simulink library "inp"  (R2021b)
settings: Solver=VariableStepAuto  StartTime=0.0  StopTime=10.0  RelTol=1e-3
undefined symbols (not defined in the file): C_TASK_5MS_S, FALSE, KINP_AcoreReadyToSlp_flg_ovrdflg, KINP_AcoreReadyToSlp_flg_ovrdval, KINP_AllowMovThd_OTA_enum_ovrdflg, KINP_AllowMovThd_OTA_enum_ovrdval, KINP_APSAngleTarget_Deg_ovrdflg, KINP_APSAngleTarget_Deg_ovrdval, KINP_APSDecReq_mps2_ovrdflg, KINP_APSDecReq_mps2_ovrdval, KINP_APSDecReqA_flg_ovrdflg, KINP_APSDecReqA_flg_ovrdval, KINP_APSDFLL_cm_ovrdflg, KINP_APSDFLL_cm_ovrdval, KINP_APSDFLR_cm_ovrdflg, KINP_APSDFLR_cm_ovrdval, KINP_APSDRLL_cm_ovrdflg, KINP_APSDRLL_cm_ovrdval, KINP_APSDRLR_cm_ovrdflg, KINP_APSDRLR_cm_ovrdval, KINP_APSExitCondition_enum_ovrdflg, KINP_APSExitCondition_enum_ovrdval, KINP_APSHWVer_enum_ovrdflg, KINP_APSHWVer_enum_ovrdval, KINP_APSProgressPCT_pct_ovrdflg, KINP_APSProgressPCT_pct_ovrdval, KINP_APSReq_enum_ovrdflg, KINP_APSReq_enum_ovrdval, KINP_APSRQDisplay_enum_ovrdflg, KINP_APSRQDisplay_enum_ovrdval, KINP_APSRqEPASCtrl_flg_ovrdflg, KINP_APSRqEPASCtrl_flg_ovrdval, KINP_APSShiftPosnReq_enum_ovrdval, KINP_APSShiftPosnReq_enum_ovrflg, KINP_APSSpeedCMD_kph_ovrdval, KINP_APSSpeedCMD_kph_ovrflg, KINP_APSStaSystem_enum_ovrdflg, KINP_APSStaSystem_enum_ovrdval, KINP_APSSWVer_enum_ovrdflg, KINP_APSSWVer_enum_ovrdval, KINP_APSVMCReqA_flg_ovrdval, KINP_APSVMCReqA_flg_ovrflg, KINP_APSVRqEPASCtrl_flg_ovrdflg, KINP_APSVRqEPASCtrl_flg_ovrdval, KINP_AuxBattVolmV_mV_ovrdflg, KINP_AuxBattVolmV_mV_ovrdval, KINP_CAASSta_enum_ovrdflg, KINP_CAASSta_enum_ovrdval, KINP_CAASVMCReqA_flg_ovrdval, KINP_CAASVMCReqA_flg_ovrflg, KINP_Chime_enum_ovrdflg, KINP_Chime_enum_ovrdval, KINP_ClearDTCcmd_flg_ovrdflg, KINP_ClearDTCcmd_flg_ovrdval, KINP_EvccAplusPwrUpReq_flg_ovrdflg, KINP_EvccAplusPwrUpReq_flg_ovrdval, KINP_LFID_raw_ovrdval, KINP_LFID_raw_ovrflg, KINP_LRID_raw_ovrdval, KINP_MemOffsetAccX_raw16_ovrdflg ... (+118)
libraries: FVT_lib x595, hcu_lib x1
(part 6 of 27)

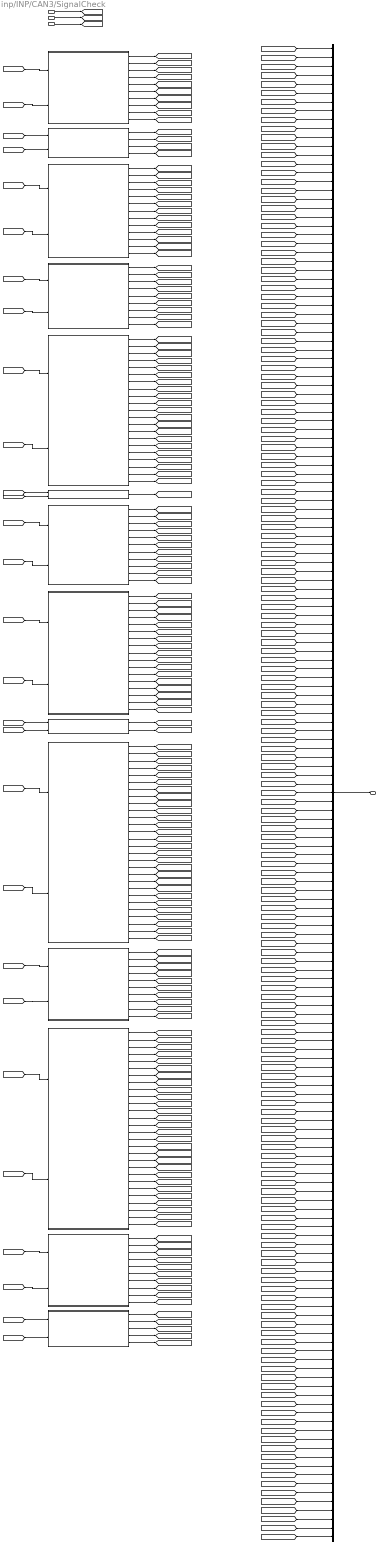
== system inp/INP/CAN3/SignalCheck ==
  inp_CanValid_bus : Inport
  TASK_TIME_S : Inport  Port=2
  BHAL_outputs : Inport  Port=3
  BMS1 : Subsystem
  BMS2 : Subsystem
  BMS3 : Subsystem
  BMS4 : Subsystem
  BMS6 : Subsystem
  BMS7 : Subsystem
  CCU1 : Subsystem
  CCU2 : Subsystem
  CCU4 : Subsystem
  MCU_F1 : Subsystem
  MCU_F2 : Subsystem
  MCU_R1 : Subsystem
  MCU_R2 : Subsystem
  Shifter1 : Subsystem
  bus_creator : BusCreator  Inputs=169
  inp_Hal_bus : Outport
  wires:
  inp_CanValid_bus/1 -> [inp_CanValid_bus]
  TASK_TIME_S/1 -> [TASK_TIME_S]
  BHAL_outputs/1 -> [BHAL_outputs]
  [BHAL_outputs] -> BMS1/1(BHAL_outputs)
  [inp_CanValid_bus] -> BMS1/2(inp_CanValid_bus)
  BMS1/1(VINP_BMS1CSErr_flg) -> [VINP_BMS1CSErr_flg]
  BMS1/2(VINP_BMS1RCErr_flg) -> [VINP_BMS1RCErr_flg]
  BMS1/3(VINP_BMSChckSum1_enum) -> [VINP_BMSChckSum1_enum]
  BMS1/4(VINP_BMSRolCnct1_enum) -> [VINP_BMSRolCnct1_enum]
  BMS1/5(VINP_HVBPwrAvailChrg_kW) -> [VINP_HVBPwrAvailChrg_kW]
  BMS1/6(VINP_HVBPwrAvailChrg30_kW) -> [VINP_HVBPwrAvailChrg30_kW]
  BMS1/7(VINP_HVBPwrAvailChrg60_kW) -> [VINP_HVBPwrAvailChrg60_kW]
  BMS1/8(VINP_HVBPwrAvailDchrg_kW) -> [VINP_HVBPwrAvailDchrg_kW]
  BMS1/9(VINP_HVBPwrAvailDchrg30_kW) -> [VINP_HVBPwrAvailDchrg30_kW]
  BMS1/10(VINP_HVBPwrAvailDchrg60_kW) -> [VINP_HVBPwrAvailDchrg60_kW]
  [BHAL_outputs] -> BMS2/1(BHAL_outputs)
  [inp_CanValid_bus] -> BMS2/2(inp_CanValid_bus)
  BMS2/1(VINP_HVInVolt_V) -> [VINP_HVInVolt_V]
  BMS2/2(VINP_LVBattDet12V_V) -> [VINP_LVBattDet12V_V]
  BMS2/3(VINP_OBCDCCurLm_A) -> [VINP_OBCDCCurLm_A]
  BMS2/4(VINP_OBCDCVoltLm_V) -> [VINP_OBCDCVoltLm_V]
  [BHAL_outputs] -> BMS3/1(BHAL_outputs)
  [inp_CanValid_bus] -> BMS3/2(inp_CanValid_bus)
  BMS3/1(VINP_ACChrgCurrDis_A) -> [VINP_ACChrgCurrDis_A]
  BMS3/2(VINP_HVBChrgPwr_kWh) -> [VINP_HVBChrgPwr_kWh]
  BMS3/3(VINP_HVBChrgPwrTotal_kWh) -> [VINP_HVBChrgPwrTotal_kWh]
  BMS3/4(VINP_HVBDrvPwr_kWh) -> [VINP_HVBDrvPwr_kWh]
  BMS3/5(VINP_HVBDrvPwrTotal_kWh) -> [VINP_HVBDrvPwrTotal_kWh]
  BMS3/6(VINP_HVBFullChrgPwr_kWh) -> [VINP_HVBFullChrgPwr_kWh]
  BMS3/7(VINP_HVBIsoImpedenceN_Megaohm) -> [VINP_HVBIsoImpedenceN_Megaohm]
  BMS3/8(VINP_HVBIsoImpedenceP_Megaohm) -> [VINP_HVBIsoImpedenceP_Megaohm]
  BMS3/9(VINP_HVBSOH_pct) -> [VINP_HVBSOH_pct]
  BMS3/10(VINP_HVBattPackVolt_V) -> [VINP_HVBattPackVolt_V]
  BMS3/11(VINP_HVBattSOC_pct) -> [VINP_HVBattSOC_pct]
  BMS3/12(VINP_HVBattSOCDis_pct) -> [VINP_HVBattSOCDis_pct]
  BMS3/13(VINP_RemainChrgTime_min) -> [VINP_RemainChrgTime_min]
  [BHAL_outputs] -> BMS4/1(BHAL_outputs)
  [inp_CanValid_bus] -> BMS4/2(inp_CanValid_bus)
  BMS4/1(VINP_CellTempAvg_C) -> [VINP_CellTempAvg_C]
  BMS4/2(VINP_HVBCellVoltMax_mV) -> [VINP_HVBCellVoltMax_mV]
  BMS4/3(VINP_HVBCellVoltMin_mV) -> [VINP_HVBCellVoltMin_mV]
  BMS4/4(VINP_HVBMTempMax_C) -> [VINP_HVBMTempMax_C]
  BMS4/5(VINP_HVBMTempMin_C) -> [VINP_HVBMTempMin_C]
  BMS4/6(VINP_MaxCellTempNum_enum) -> [VINP_MaxCellTempNum_enum]
  BMS4/7(VINP_MaxCellVoltNum_enum) -> [VINP_MaxCellVoltNum_enum]
  BMS4/8(VINP_MinCellTempNum_enum) -> [VINP_MinCellTempNum_enum]
  BMS4/9(VINP_MinCellVoltNum_enum) -> [VINP_MinCellVoltNum_enum]
  [BHAL_outputs] -> BMS6/1(BHAL_outputs)
  [inp_CanValid_bus] -> BMS6/2(inp_CanValid_bus)
  BMS6/1(VINP_BMS6CSErr_flg) -> [VINP_BMS6CSErr_flg]
  BMS6/2(VINP_BMS6RCErr_flg) -> [VINP_BMS6RCErr_flg]
  BMS6/3(VINP_BMSChckSum_enum) -> [VINP_BMSChckSum_enum]
  BMS6/4(VINP_BMSRolCnct_enum) -> [VINP_BMSRolCnct_enum]
  BMS6/5(VINP_BMSREADY_flg) -> [VINP_BMSREADY_flg]
  BMS6/6(VINP_BMSWarn1_flg) -> [VINP_BMSWarn1_flg]
  BMS6/7(VINP_BMSWarn2_flg) -> [VINP_BMSWarn2_flg]
  BMS6/8(VINP_BMSWarn3_flg) -> [VINP_BMSWarn3_flg]
  BMS6/9(VINP_BMSWarn4_flg) -> [VINP_BMSWarn4_flg]
  BMS6/10(VINP_BMSWarn5_flg) -> [VINP_BMSWarn5_flg]
  BMS6/11(VINP_BMSWarn6_flg) -> [VINP_BMSWarn6_flg]
  BMS6/12(VINP_BMSWarn7_flg) -> [VINP_BMSWarn7_flg]
  BMS6/13(VINP_BMSWarn8_flg) -> [VINP_BMSWarn8_flg]
  BMS6/14(VINP_ChrgPlugSta_enum) -> [VINP_ChrgPlugSta_enum]
  BMS6/15(VINP_ExtChrgSta_enum) -> [VINP_ExtChrgSta_enum]
  BMS6/16(VINP_HVBContactorSta_flg) -> [VINP_HVBContactorSta_flg]
  BMS6/17(VINP_HVBHVILErr_flg) -> [VINP_HVBHVILErr_flg]
  BMS6/18(VINP_HVBPreheatPrecoolSta_enum) -> [VINP_HVBPreheatPrecoolSta_enum]
  BMS6/19(VINP_HVBattReady4Pre_enum) -> [VINP_HVBattReady4Pre_enum]
  BMS6/20(VINP_HVILSta_flg) -> [VINP_HVILSta_flg]
  BMS6/21(VINP_V2LSta_enum) -> [VINP_V2LSta_enum]
  [BHAL_outputs] -> BMS7/1(BHAL_outputs)
  [inp_CanValid_bus] -> BMS7/2(inp_CanValid_bus)
  BMS7/1(VINP_HVBattErr_flg) -> [VINP_HVBattErr_flg]
  [BHAL_outputs] -> CCU1/1(BHAL_outputs)
  [inp_CanValid_bus] -> CCU1/2(inp_CanValid_bus)
  CCU1/1(VINP_CCU1CSErr_flg) -> [VINP_CCU1CSErr_flg]
  CCU1/2(VINP_CCU1RCErr_flg) -> [VINP_CCU1RCErr_flg]
  CCU1/3(VINP_CSCCU1_enum) -> [VINP_CSCCU1_enum]
  CCU1/4(VINP_DCDCAuxVolt_V) -> [VINP_DCDCAuxVolt_V]
  CCU1/5(VINP_DCDCInVoltInf_V) -> [VINP_DCDCInVoltInf_V]
  CCU1/6(VINP_DCDCPreCompleted_enum) -> [VINP_DCDCPreCompleted_enum]
  CCU1/7(VINP_OBCDCCurrInf_A) -> [VINP_OBCDCCurrInf_A]
  CCU1/8(VINP_OBCDCVoltInf_V) -> [VINP_OBCDCVoltInf_V]
  CCU1/9(VINP_OBCPreCompleted_enum) -> [VINP_OBCPreCompleted_enum]
  CCU1/10(VINP_OBCWakeup4Plugin_flg) -> [VINP_OBCWakeup4Plugin_flg]
  CCU1/11(VINP_RCCCU1_enum) -> [VINP_RCCCU1_enum]
  [BHAL_outputs] -> CCU2/1(BHAL_outputs)
  [inp_CanValid_bus] -> CCU2/2(inp_CanValid_bus)
  CCU2/1(VINP_CCU2CSErr_flg) -> [VINP_CCU2CSErr_flg]
  CCU2/2(VINP_CCU2RCErr_flg) -> [VINP_CCU2RCErr_flg]
  CCU2/3(VINP_CSCCU2_enum) -> [VINP_CSCCU2_enum]
  CCU2/4(VINP_DCDCEnaSta_flg) -> [VINP_DCDCEnaSta_flg]
  CCU2/5(VINP_DCDCFaultSta_enum) -> [VINP_DCDCFaultSta_enum]
  CCU2/6(VINP_DCDCReady4Pre_flg) -> [VINP_DCDCReady4Pre_flg]
  CCU2/7(VINP_DCDCTemp_C) -> [VINP_DCDCTemp_C]
  CCU2/8(VINP_OBCACCurrInf_A) -> [VINP_OBCACCurrInf_A]
  CCU2/9(VINP_OBCACVoltInf_V) -> [VINP_OBCACVoltInf_V]
  CCU2/10(VINP_OBCEnaSta_flg) -> [VINP_OBCEnaSta_flg]
  CCU2/11(VINP_OBCFaultSta_enum) -> [VINP_OBCFaultSta_enum]
  CCU2/12(VINP_OBCPluginSta_flg) -> [VINP_OBCPluginSta_flg]
  CCU2/13(VINP_OBCReady4Pre_flg) -> [VINP_OBCReady4Pre_flg]
  CCU2/14(VINP_OBCTemp_C) -> [VINP_OBCTemp_C]
  CCU2/15(VINP_OBCV2LSta_enum) -> [VINP_OBCV2LSta_enum]
  CCU2/16(VINP_OBCACCurLim_enum) -> [VINP_OBCACCurLim_enum]
  CCU2/17(VINP_RCCCU2_enum) -> [VINP_RCCCU2_enum]
  [BHAL_outputs] -> CCU4/1(BHAL_outputs)
  [inp_CanValid_bus] -> CCU4/2(inp_CanValid_bus)
  CCU4/1(VINP_DCDCAuxCur_A) -> [VINP_DCDCAuxCur_A]
  CCU4/2(VINP_DCDCHVCur_A) -> [VINP_DCDCHVCur_A]
  [BHAL_outputs] -> MCU_F1/1(BHAL_outputs)
  [inp_CanValid_bus] -> MCU_F1/2(inp_CanValid_bus)
  MCU_F1/1(VINP_MCUF1CSErr_flg) -> [VINP_MCUF1CSErr_flg]
  MCU_F1/2(VINP_MCUF1RCErr_flg) -> [VINP_MCUF1RCErr_flg]
  MCU_F1/3(VINP_FrActvDmpDisabSta_flg) -> [VINP_FrActvDmpDisabSta_flg]
  MCU_F1/4(VINP_FrEDUDrtSta_flg) -> [VINP_FrEDUDrtSta_flg]
  MCU_F1/5(VINP_FrEDUOpratingSta_flg) -> [VINP_FrEDUOpratingSta_flg]
  MCU_F1/6(VINP_FrEDURealTMTq_Nm) -> [VINP_FrEDURealTMTq_Nm]
  MCU_F1/7(VINP_FrEDURotateDirction_enum) -> [VINP_FrEDURotateDirction_enum]
  MCU_F1/8(VINP_FrEDUTqReqFbk_Nm) -> [VINP_FrEDUTqReqFbk_Nm]
  MCU_F1/9(VINP_FrMCU1Chksum_enum) -> [VINP_FrMCU1Chksum_enum]
  MCU_F1/10(VINP_FrMCU1RolCnt_enum) -> [VINP_FrMCU1RolCnt_enum]
  MCU_F1/11(VINP_FrMCUBAT_V) -> [VINP_FrMCUBAT_V]
  MCU_F1/12(VINP_FrMCUDCBusCurr_A) -> [VINP_FrMCUDCBusCurr_A]
  MCU_F1/13(VINP_FrMCUDCBusVolt_V) -> [VINP_FrMCUDCBusVolt_V]
  MCU_F1/14(VINP_FrMCUDischrgSta_flg) -> [VINP_FrMCUDischrgSta_flg]
  MCU_F1/15(VINP_FrMCUEnaSta_flg) -> [VINP_FrMCUEnaSta_flg]
  MCU_F1/16(VINP_FrMCUErr_enum) -> [VINP_FrMCUErr_enum]
  MCU_F1/17(VINP_FrMCUIGNsta_flg) -> [VINP_FrMCUIGNsta_flg]
  MCU_F1/18(VINP_FrMCUReady_flg) -> [VINP_FrMCUReady_flg]
  MCU_F1/19(VINP_FrMCUReady4Pre_flg) -> [VINP_FrMCUReady4Pre_flg]
  MCU_F1/20(VINP_FrMCUSysSta_enum) -> [VINP_FrMCUSysSta_enum]
  MCU_F1/21(VINP_FrMCUTemp_C) -> [VINP_FrMCUTemp_C]
  MCU_F1/22(VINP_FrMotorAvailTq_Nm) -> [VINP_FrMotorAvailTq_Nm]
  MCU_F1/23(VINP_FrRegenAvailTq_Nm) -> [VINP_FrRegenAvailTq_Nm]
  MCU_F1/24(VINP_FrTMSpd_rpm) -> [VINP_FrTMSpd_rpm]
  MCU_F1/25(VINP_FrTMTemp_C) -> [VINP_FrTMTemp_C]
  MCU_F1/26(VINP_FrTMid_A) -> [VINP_FrTMid_A]
  MCU_F1/27(VINP_FrTMiq_A) -> [VINP_FrTMiq_A]
  MCU_F1/28(VINP_MCUWarnF_enum) -> [VINP_MCUWarnF_enum]
  [BHAL_outputs] -> MCU_F2/1(BHAL_outputs)
  [inp_CanValid_bus] -> MCU_F2/2(inp_CanValid_bus)
  MCU_F2/1(VINP_FrCoolanttempReq_C) -> [VINP_FrCoolanttempReq_C]
  MCU_F2/2(VINP_FrEOPSpdSet_rpm) -> [VINP_FrEOPSpdSet_rpm]
  MCU_F2/3(VINP_FrFailcode1_enum) -> [VINP_FrFailcode1_enum]
  MCU_F2/4(VINP_FrFailcode2_enum) -> [VINP_FrFailcode2_enum]
  MCU_F2/5(VINP_FrFailcodehistory1_enum) -> [VINP_FrFailcodehistory1_enum]
  MCU_F2/6(VINP_FrFailcodehistory2_enum) -> [VINP_FrFailcodehistory2_enum]
  MCU_F2/7(VINP_FrLLCTemp_C) -> [VINP_FrLLCTemp_C]
  MCU_F2/8(VINP_FrLLCflowReq_Lpmin) -> [VINP_FrLLCflowReq_Lpmin]
  MCU_F2/9(VINP_FrMCUTempWarn_enum) -> [VINP_FrMCUTempWarn_enum]
  MCU_F2/10(VINP_FrTMTempWarn_enum) -> [VINP_FrTMTempWarn_enum]
  [BHAL_outputs] -> MCU_R1/1(BHAL_outputs)
  [inp_CanValid_bus] -> MCU_R1/2(inp_CanValid_bus)
  MCU_R1/1(VINP_MCUR1CSErr_flg) -> [VINP_MCUR1CSErr_flg]
  MCU_R1/2(VINP_MCUR1RCErr_flg) -> [VINP_MCUR1RCErr_flg]
  MCU_R1/3(VINP_MCUWarnR_enum) -> [VINP_MCUWarnR_enum]
  MCU_R1/4(VINP_RrActvDmpDisabSta_flg) -> [VINP_RrActvDmpDisabSta_flg]
  MCU_R1/5(VINP_RrEDUDrtSta_flg) -> [VINP_RrEDUDrtSta_flg]
  MCU_R1/6(VINP_RrEDUOpratingSta_flg) -> [VINP_RrEDUOpratingSta_flg]
  MCU_R1/7(VINP_RrEDURealTMTq_Nm) -> [VINP_RrEDURealTMTq_Nm]
  MCU_R1/8(VINP_RrEDURotateDirction_enum) -> [VINP_RrEDURotateDirction_enum]
  MCU_R1/9(VINP_RrEDUTqReqFbk_Nm) -> [VINP_RrEDUTqReqFbk_Nm]
  MCU_R1/10(VINP_RrMCU1Chksum_enum) -> [VINP_RrMCU1Chksum_enum]
  MCU_R1/11(VINP_RrMCU1RolCnt_enum) -> [VINP_RrMCU1RolCnt_enum]
  MCU_R1/12(VINP_RrMCUBAT_V) -> [VINP_RrMCUBAT_V]
  MCU_R1/13(VINP_RrMCUDCBusCurr_A) -> [VINP_RrMCUDCBusCurr_A]
  MCU_R1/14(VINP_RrMCUDCBusVolt_V) -> [VINP_RrMCUDCBusVolt_V]
  MCU_R1/15(VINP_RrMCUDischrgSta_flg) -> [VINP_RrMCUDischrgSta_flg]
  MCU_R1/16(VINP_RrMCUEnaSta_flg) -> [VINP_RrMCUEnaSta_flg]
  MCU_R1/17(VINP_RrMCUErr_enum) -> [VINP_RrMCUErr_enum]
  MCU_R1/18(VINP_RrMCUIGNsta_flg) -> [VINP_RrMCUIGNsta_flg]
  MCU_R1/19(VINP_RrMCUReady_flg) -> [VINP_RrMCUReady_flg]
  MCU_R1/20(VINP_RrMCUReady4Pre_flg) -> [VINP_RrMCUReady4Pre_flg]
  MCU_R1/21(VINP_RrMCUSysSta_enum) -> [VINP_RrMCUSysSta_enum]
  MCU_R1/22(VINP_RrMCUTemp_C) -> [VINP_RrMCUTemp_C]
  MCU_R1/23(VINP_RrMotorAvailTq_Nm) -> [VINP_RrMotorAvailTq_Nm]
  MCU_R1/24(VINP_RrRegenAvailTq_Nm) -> [VINP_RrRegenAvailTq_Nm]
  MCU_R1/25(VINP_RrTMSpd_rpm) -> [VINP_RrTMSpd_rpm]
  MCU_R1/26(VINP_RrTMTemp_C) -> [VINP_RrTMTemp_C]
  MCU_R1/27(VINP_RrTMid_A) -> [VINP_RrTMid_A]
  MCU_R1/28(VINP_RrTMiq_A) -> [VINP_RrTMiq_A]
  [BHAL_outputs] -> MCU_R2/1(BHAL_outputs)
  [inp_CanValid_bus] -> MCU_R2/2(inp_CanValid_bus)
  MCU_R2/1(VINP_RrCoolanttempReq_cnt) -> [VINP_RrCoolanttempReq_cnt]
  MCU_R2/2(VINP_RrEOPSpdSet_rpm) -> [VINP_RrEOPSpdSet_rpm]
  MCU_R2/3(VINP_RrFailcode1_enum) -> [VINP_RrFailcode1_enum]
  MCU_R2/4(VINP_RrFailcode2_enum) -> [VINP_RrFailcode2_enum]
  MCU_R2/5(VINP_RrFailcodehistory1_enum) -> [VINP_RrFailcodehistory1_enum]
  MCU_R2/6(VINP_RrFailcodehistory2_enum) -> [VINP_RrFailcodehistory2_enum]
  MCU_R2/7(VINP_RrLLCTemp_C) -> [VINP_RrLLCTemp_C]
  MCU_R2/8(VINP_RrLLCflowReq_Lpmin) -> [VINP_RrLLCflowReq_Lpmin]
  MCU_R2/9(VINP_RrMCUTempWarn_enum) -> [VINP_RrMCUTempWarn_enum]
  MCU_R2/10(VINP_RrTMTempWarn_enum) -> [VINP_RrTMTempWarn_enum]
  [BHAL_outputs] -> Shifter1/1(BHAL_outputs)
  [inp_CanValid_bus] -> Shifter1/2(inp_CanValid_bus)
  Shifter1/1(VINP_Shifter1CSErr_flg) -> [VINP_Shifter1CSErr_flg]
  Shifter1/2(VINP_Shifter1RCErr_flg) -> [VINP_Shifter1RCErr_flg]
  Shifter1/3(VINP_ShifterCRC8_enum) -> [VINP_ShifterCRC8_enum]
  Shifter1/4(VINP_ShifterHandleCmd_enum) -> [VINP_ShifterHandleCmd_enum]
  Shifter1/5(VINP_ShifterRC_enum) -> [VINP_ShifterRC_enum]
  bus_creator/1 -> inp_Hal_bus/1
  [VINP_BMS1CSErr_flg] -> bus_creator/1
  [VINP_BMS1RCErr_flg] -> bus_creator/2
  [VINP_BMSChckSum1_enum] -> bus_creator/3
  [VINP_BMSRolCnct1_enum] -> bus_creator/4
  [VINP_HVBPwrAvailChrg_kW] -> bus_creator/5
  [VINP_HVBPwrAvailChrg30_kW] -> bus_creator/6
  [VINP_HVBPwrAvailChrg60_kW] -> bus_creator/7
  [VINP_HVBPwrAvailDchrg_kW] -> bus_creator/8
  [VINP_HVBPwrAvailDchrg30_kW] -> bus_creator/9
  [VINP_HVBPwrAvailDchrg60_kW] -> bus_creator/10
  [VINP_HVInVolt_V] -> bus_creator/11
  [VINP_LVBattDet12V_V] -> bus_creator/12
  [VINP_OBCDCCurLm_A] -> bus_creator/13
  [VINP_OBCDCVoltLm_V] -> bus_creator/14
  [VINP_ACChrgCurrDis_A] -> bus_creator/15
  [VINP_HVBChrgPwr_kWh] -> bus_creator/16
  [VINP_HVBChrgPwrTotal_kWh] -> bus_creator/17
  [VINP_HVBDrvPwr_kWh] -> bus_creator/18
  [VINP_HVBDrvPwrTotal_kWh] -> bus_creator/19
  [VINP_HVBFullChrgPwr_kWh] -> bus_creator/20
  [VINP_HVBIsoImpedenceN_Megaohm] -> bus_creator/21
  [VINP_HVBIsoImpedenceP_Megaohm] -> bus_creator/22
  [VINP_HVBSOH_pct] -> bus_creator/23
  [VINP_HVBattPackVolt_V] -> bus_creator/24
  [VINP_HVBattSOC_pct] -> bus_creator/25
  [VINP_HVBattSOCDis_pct] -> bus_creator/26
  [VINP_RemainChrgTime_min] -> bus_creator/27
  [VINP_CellTempAvg_C] -> bus_creator/28
  [VINP_HVBCellVoltMax_mV] -> bus_creator/29
  [VINP_HVBCellVoltMin_mV] -> bus_creator/30
  [VINP_HVBMTempMax_C] -> bus_creator/31
  [VINP_HVBMTempMin_C] -> bus_creator/32
  [VINP_MaxCellTempNum_enum] -> bus_creator/33
  [VINP_MaxCellVoltNum_enum] -> bus_creator/34
  [VINP_MinCellTempNum_enum] -> bus_creator/35
  [VINP_MinCellVoltNum_enum] -> bus_creator/36
  [VINP_BMS6CSErr_flg] -> bus_creator/37
  [VINP_BMS6RCErr_flg] -> bus_creator/38
  [VINP_BMSChckSum_enum] -> bus_creator/39
  [VINP_BMSRolCnct_enum] -> bus_creator/40
  [VINP_BMSREADY_flg] -> bus_creator/41
  [VINP_BMSWarn1_flg] -> bus_creator/42
  [VINP_BMSWarn2_flg] -> bus_creator/43
  [VINP_BMSWarn3_flg] -> bus_creator/44
  [VINP_BMSWarn4_flg] -> bus_creator/45
  [VINP_BMSWarn5_flg] -> bus_creator/46
  [VINP_BMSWarn6_flg] -> bus_creator/47
  [VINP_BMSWarn7_flg] -> bus_creator/48
  [VINP_BMSWarn8_flg] -> bus_creator/49
  [VINP_ChrgPlugSta_enum] -> bus_creator/50
  [VINP_ExtChrgSta_enum] -> bus_creator/51
  [VINP_HVBContactorSta_flg] -> bus_creator/52
  [VINP_HVBHVILErr_flg] -> bus_creator/53
  [VINP_HVBPreheatPrecoolSta_enum] -> bus_creator/54
  [VINP_HVBattReady4Pre_enum] -> bus_creator/55
  [VINP_HVILSta_flg] -> bus_creator/56
  [VINP_V2LSta_enum] -> bus_creator/57
  [VINP_HVBattErr_flg] -> bus_creator/58
  [VINP_CCU1CSErr_flg] -> bus_creator/59
  [VINP_CCU1RCErr_flg] -> bus_creator/60
  [VINP_CSCCU1_enum] -> bus_creator/61
  [VINP_DCDCAuxVolt_V] -> bus_creator/62
  [VINP_DCDCInVoltInf_V] -> bus_creator/63
  [VINP_DCDCPreCompleted_enum] -> bus_creator/64
  [VINP_OBCDCCurrInf_A] -> bus_creator/65
  [VINP_OBCDCVoltInf_V] -> bus_creator/66
  [VINP_OBCPreCompleted_enum] -> bus_creator/67
  [VINP_OBCWakeup4Plugin_flg] -> bus_creator/68
  [VINP_RCCCU1_enum] -> bus_creator/69
  [VINP_CCU2CSErr_flg] -> bus_creator/70
  [VINP_CCU2RCErr_flg] -> bus_creator/71
  [VINP_CSCCU2_enum] -> bus_creator/72
  [VINP_DCDCEnaSta_flg] -> bus_creator/73
  [VINP_DCDCFaultSta_enum] -> bus_creator/74
  [VINP_DCDCReady4Pre_flg] -> bus_creator/75
  [VINP_DCDCTemp_C] -> bus_creator/76
  [VINP_OBCACCurrInf_A] -> bus_creator/77
  [VINP_OBCACVoltInf_V] -> bus_creator/78
  [VINP_OBCEnaSta_flg] -> bus_creator/79
  [VINP_OBCFaultSta_enum] -> bus_creator/80
  [VINP_OBCPluginSta_flg] -> bus_creator/81
  [VINP_OBCReady4Pre_flg] -> bus_creator/82
  [VINP_OBCTemp_C] -> bus_creator/83
  [VINP_OBCV2LSta_enum] -> bus_creator/84
  [VINP_OBCACCurLim_enum] -> bus_creator/85
  [VINP_RCCCU2_enum] -> bus_creator/86
  [VINP_DCDCAuxCur_A] -> bus_creator/87
  [VINP_DCDCHVCur_A] -> bus_creator/88
  [VINP_MCUF1CSErr_flg] -> bus_creator/89
  [VINP_MCUF1RCErr_flg] -> bus_creator/90
  [VINP_FrActvDmpDisabSta_flg] -> bus_creator/91
  [VINP_FrEDUDrtSta_flg] -> bus_creator/92
  [VINP_FrEDUOpratingSta_flg] -> bus_creator/93
  [VINP_FrEDURealTMTq_Nm] -> bus_creator/94
  [VINP_FrEDURotateDirction_enum] -> bus_creator/95
  [VINP_FrEDUTqReqFbk_Nm] -> bus_creator/96
  [VINP_FrMCU1Chksum_enum] -> bus_creator/97
  [VINP_FrMCU1RolCnt_enum] -> bus_creator/98
  [VINP_FrMCUBAT_V] -> bus_creator/99
  [VINP_FrMCUDCBusCurr_A] -> bus_creator/100
  [VINP_FrMCUDCBusVolt_V] -> bus_creator/101
  [VINP_FrMCUDischrgSta_flg] -> bus_creator/102
  [VINP_FrMCUEnaSta_flg] -> bus_creator/103
  [VINP_FrMCUErr_enum] -> bus_creator/104
  [VINP_FrMCUIGNsta_flg] -> bus_creator/105
  [VINP_FrMCUReady_flg] -> bus_creator/106
  [VINP_FrMCUReady4Pre_flg] -> bus_creator/107
  [VINP_FrMCUSysSta_enum] -> bus_creator/108
  [VINP_FrMCUTemp_C] -> bus_creator/109
  [VINP_FrMotorAvailTq_Nm] -> bus_creator/110
  [VINP_FrRegenAvailTq_Nm] -> bus_creator/111
  [VINP_FrTMSpd_rpm] -> bus_creator/112
  [VINP_FrTMTemp_C] -> bus_creator/113
  [VINP_FrTMid_A] -> bus_creator/114
  [VINP_FrTMiq_A] -> bus_creator/115
  [VINP_MCUWarnF_enum] -> bus_creator/116
  [VINP_FrCoolanttempReq_C] -> bus_creator/117
  [VINP_FrEOPSpdSet_rpm] -> bus_creator/118
  [VINP_FrFailcode1_enum] -> bus_creator/119
  [VINP_FrFailcode2_enum] -> bus_creator/120
  [VINP_FrFailcodehistory1_enum] -> bus_creator/121
  [VINP_FrFailcodehistory2_enum] -> bus_creator/122
  [VINP_FrLLCTemp_C] -> bus_creator/123
  [VINP_FrLLCflowReq_Lpmin] -> bus_creator/124
  [VINP_FrMCUTempWarn_enum] -> bus_creator/125
  [VINP_FrTMTempWarn_enum] -> bus_creator/126
  [VINP_MCUR1CSErr_flg] -> bus_creator/127
  [VINP_MCUR1RCErr_flg] -> bus_creator/128
  [VINP_MCUWarnR_enum] -> bus_creator/129
  [VINP_RrActvDmpDisabSta_flg] -> bus_creator/130
  [VINP_RrEDUDrtSta_flg] -> bus_creator/131
  [VINP_RrEDUOpratingSta_flg] -> bus_creator/132
  [VINP_RrEDURealTMTq_Nm] -> bus_creator/133
  [VINP_RrEDURotateDirction_enum] -> bus_creator/134
  [VINP_RrEDUTqReqFbk_Nm] -> bus_creator/135
  [VINP_RrMCU1Chksum_enum] -> bus_creator/136
  [VINP_RrMCU1RolCnt_enum] -> bus_creator/137
  [VINP_RrMCUBAT_V] -> bus_creator/138
  [VINP_RrMCUDCBusCurr_A] -> bus_creator/139
  [VINP_RrMCUDCBusVolt_V] -> bus_creator/140
  [VINP_RrMCUDischrgSta_flg] -> bus_creator/141
  [VINP_RrMCUEnaSta_flg] -> bus_creator/142
  [VINP_RrMCUErr_enum] -> bus_creator/143
  [VINP_RrMCUIGNsta_flg] -> bus_creator/144
  [VINP_RrMCUReady_flg] -> bus_creator/145
  [VINP_RrMCUReady4Pre_flg] -> bus_creator/146
  [VINP_RrMCUSysSta_enum] -> bus_creator/147
  [VINP_RrMCUTemp_C] -> bus_creator/148
  [VINP_RrMotorAvailTq_Nm] -> bus_creator/149
  [VINP_RrRegenAvailTq_Nm] -> bus_creator/150
  [VINP_RrTMSpd_rpm] -> bus_creator/151
  [VINP_RrTMTemp_C] -> bus_creator/152
  [VINP_RrTMid_A] -> bus_creator/153
  [VINP_RrTMiq_A] -> bus_creator/154
  [VINP_RrCoolanttempReq_cnt] -> bus_creator/155
  [VINP_RrEOPSpdSet_rpm] -> bus_creator/156
  [VINP_RrFailcode1_enum] -> bus_creator/157
  [VINP_RrFailcode2_enum] -> bus_creator/158
  [VINP_RrFailcodehistory1_enum] -> bus_creator/159
  [VINP_RrFailcodehistory2_enum] -> bus_creator/160
  [VINP_RrLLCTemp_C] -> bus_creator/161
  [VINP_RrLLCflowReq_Lpmin] -> bus_creator/162
  [VINP_RrMCUTempWarn_enum] -> bus_creator/163
  [VINP_RrTMTempWarn_enum] -> bus_creator/164
  [VINP_Shifter1CSErr_flg] -> bus_creator/165
  [VINP_Shifter1RCErr_flg] -> bus_creator/166
  [VINP_ShifterCRC8_enum] -> bus_creator/167
  [VINP_ShifterHandleCmd_enum] -> bus_creator/168
  [VINP_ShifterRC_enum] -> bus_creator/169

== system inp/INP/CAN4/CommunicationCheck ==
  BHAL_outputs : Inport
  CANMsgInvalidDKC1 : FVT_lib/inp/CAN_Msg_Validity_Process_template  SystemSampleTime=-1  VariantActivationTime=update diagram  Latency=0  AutoFrameSizeCalculation=off
      link override debdec: Value=KINP_CANMsgInvalidDKC1_flg_debdec
      link override debinc: Value=KINP_CANMsgInvalidDKC1_flg_debinc
      link override deblim: Value=KINP_CANMsgInvalidDKC1_flg_deblim
      link override inverse: Value=KINP_CANMsgInvalidDKC1_flg_inverse
      link override ovrdflg: Value=KINP_CANMsgInvalidDKC1_flg_ovrdflg
      link override ovrdval: Value=KINP_CANMsgInvalidDKC1_flg_ovrdval
      link override srvcflg: Value=KINP_CANMsgInvalidDKC1_flg_srvcflg
      link override srvcval: Value=KINP_CANMsgInvalidDKC1_flg_srvcval
  CANMsgInvalidDKC2 : FVT_lib/inp/CAN_Msg_Validity_Process_template  SystemSampleTime=-1  VariantActivationTime=update diagram  Latency=0  AutoFrameSizeCalculation=off
      link override debdec: Value=KINP_CANMsgInvalidDKC2_flg_debdec
      link override debinc: Value=KINP_CANMsgInvalidDKC2_flg_debinc
      link override deblim: Value=KINP_CANMsgInvalidDKC2_flg_deblim
      link override inverse: Value=KINP_CANMsgInvalidDKC2_flg_inverse
      link override ovrdflg: Value=KINP_CANMsgInvalidDKC2_flg_ovrdflg
      link override ovrdval: Value=KINP_CANMsgInvalidDKC2_flg_ovrdval
      link override srvcflg: Value=KINP_CANMsgInvalidDKC2_flg_srvcflg
      link override srvcval: Value=KINP_CANMsgInvalidDKC2_flg_srvcval
  CANMsgInvalidGWZDRPTG1 : FVT_lib/inp/CAN_Msg_Validity_Process_template  SystemSampleTime=-1  VariantActivationTime=update diagram  Latency=0  AutoFrameSizeCalculation=off
      link override debdec: Value=KINP_CANMsgInvalidGWZDRPTG1_flg_debdec
      link override debinc: Value=KINP_CANMsgInvalidGWZDRPTG1_flg_debinc
      link override deblim: Value=KINP_CANMsgInvalidGWZDRPTG1_flg_deblim
      link override inverse: Value=KINP_CANMsgInvalidGWZDRPTG1_flg_inverse
      link override ovrdflg: Value=KINP_CANMsgInvalidGWZDRPTG1_flg_ovrdflg
      link override ovrdval: Value=KINP_CANMsgInvalidGWZDRPTG1_flg_ovrdval
      link override srvcflg: Value=KINP_CANMsgInvalidGWZDRPTG1_flg_srvcflg
      link override srvcval: Value=KINP_CANMsgInvalidGWZDRPTG1_flg_srvcval
  CANMsgInvalidGWZoneDR1 : FVT_lib/inp/CAN_Msg_Validity_Process_template  SystemSampleTime=-1  VariantActivationTime=update diagram  Latency=0  AutoFrameSizeCalculation=off
      link override debdec: Value=KINP_CANMsgInvalidGWZoneDR1_flg_debdec
      link override debinc: Value=KINP_CANMsgInvalidGWZoneDR1_flg_debinc
      link override deblim: Value=KINP_CANMsgInvalidGWZoneDR1_flg_deblim
      link override inverse: Value=KINP_CANMsgInvalidGWZoneDR1_flg_inverse
      link override ovrdflg: Value=KINP_CANMsgInvalidGWZoneDR1_flg_ovrdflg
      link override ovrdval: Value=KINP_CANMsgInvalidGWZoneDR1_flg_ovrdval
      link override srvcflg: Value=KINP_CANMsgInvalidGWZoneDR1_flg_srvcflg
      link override srvcval: Value=KINP_CANMsgInvalidGWZoneDR1_flg_srvcval
  CANMsgInvalidGWZoneDR2 : FVT_lib/inp/CAN_Msg_Validity_Process_template  SystemSampleTime=-1  VariantActivationTime=update diagram  Latency=0  AutoFrameSizeCalculation=off
      link override debdec: Value=KINP_CANMsgInvalidGWZoneDR2_flg_debdec
      link override debinc: Value=KINP_CANMsgInvalidGWZoneDR2_flg_debinc
      link override deblim: Value=KINP_CANMsgInvalidGWZoneDR2_flg_deblim
      link override inverse: Value=KINP_CANMsgInvalidGWZoneDR2_flg_inverse
      link override ovrdflg: Value=KINP_CANMsgInvalidGWZoneDR2_flg_ovrdflg
      link override ovrdval: Value=KINP_CANMsgInvalidGWZoneDR2_flg_ovrdval
      link override srvcflg: Value=KINP_CANMsgInvalidGWZoneDR2_flg_srvcflg
      link override srvcval: Value=KINP_CANMsgInvalidGWZoneDR2_flg_srvcval
  CANMsgInvalidGWZoneDR3 : FVT_lib/inp/CAN_Msg_Validity_Process_template  SystemSampleTime=-1  VariantActivationTime=update diagram  Latency=0  AutoFrameSizeCalculation=off
      link override debdec: Value=KINP_CANMsgInvalidGWZoneDR3_flg_debdec
      link override debinc: Value=KINP_CANMsgInvalidGWZoneDR3_flg_debinc
      link override deblim: Value=KINP_CANMsgInvalidGWZoneDR3_flg_deblim
      link override inverse: Value=KINP_CANMsgInvalidGWZoneDR3_flg_inverse
      link override ovrdflg: Value=KINP_CANMsgInvalidGWZoneDR3_flg_ovrdflg
      link override ovrdval: Value=KINP_CANMsgInvalidGWZoneDR3_flg_ovrdval
      link override srvcflg: Value=KINP_CANMsgInvalidGWZoneDR3_flg_srvcflg
      link override srvcval: Value=KINP_CANMsgInvalidGWZoneDR3_flg_srvcval
  CANMsgInvalidGWZoneDR4 : FVT_lib/inp/CAN_Msg_Validity_Process_template  SystemSampleTime=-1  VariantActivationTime=update diagram  Latency=0  AutoFrameSizeCalculation=off
      link override debdec: Value=KINP_CANMsgInvalidGWZoneDR4_flg_debdec
      link override debinc: Value=KINP_CANMsgInvalidGWZoneDR4_flg_debinc
      link override deblim: Value=KINP_CANMsgInvalidGWZoneDR4_flg_deblim
      link override inverse: Value=KINP_CANMsgInvalidGWZoneDR4_flg_inverse
      link override ovrdflg: Value=KINP_CANMsgInvalidGWZoneDR4_flg_ovrdflg
      link override ovrdval: Value=KINP_CANMsgInvalidGWZoneDR4_flg_ovrdval
      link override srvcflg: Value=KINP_CANMsgInvalidGWZoneDR4_flg_srvcflg
      link override srvcval: Value=KINP_CANMsgInvalidGWZoneDR4_flg_srvcval
  CANMsgInvalidGWZoneDR6 : FVT_lib/inp/CAN_Msg_Validity_Process_template  SystemSampleTime=-1  VariantActivationTime=update diagram  Latency=0  AutoFrameSizeCalculation=off
      link override debdec: Value=KINP_CANMsgInvalidGWZoneDR6_flg_debdec
      link override debinc: Value=KINP_CANMsgInvalidGWZoneDR6_flg_debinc
      link override deblim: Value=KINP_CANMsgInvalidGWZoneDR6_flg_deblim
      link override inverse: Value=KINP_CANMsgInvalidGWZoneDR6_flg_inverse
      link override ovrdflg: Value=KINP_CANMsgInvalidGWZoneDR6_flg_ovrdflg
      link override ovrdval: Value=KINP_CANMsgInvalidGWZoneDR6_flg_ovrdval
      link override srvcflg: Value=KINP_CANMsgInvalidGWZoneDR6_flg_srvcflg
      link override srvcval: Value=KINP_CANMsgInvalidGWZoneDR6_flg_srvcval
  CANMsgInvalidGWZoneFR1 : FVT_lib/inp/CAN_Msg_Validity_Process_template  SystemSampleTime=-1  VariantActivationTime=update diagram  Latency=0  AutoFrameSizeCalculation=off
      link override debdec: Value=KINP_CANMsgInvalidGWZoneFR1_flg_debdec
      link override debinc: Value=KINP_CANMsgInvalidGWZoneFR1_flg_debinc
      link override deblim: Value=KINP_CANMsgInvalidGWZoneFR1_flg_deblim
      link override inverse: Value=KINP_CANMsgInvalidGWZoneFR1_flg_inverse
      link override ovrdflg: Value=KINP_CANMsgInvalidGWZoneFR1_flg_ovrdflg
      link override ovrdval: Value=KINP_CANMsgInvalidGWZoneFR1_flg_ovrdval
      link override srvcflg: Value=KINP_CANMsgInvalidGWZoneFR1_flg_srvcflg
      link override srvcval: Value=KINP_CANMsgInvalidGWZoneFR1_flg_srvcval
  CANMsgInvalidGWZoneFR2 : FVT_lib/inp/CAN_Msg_Validity_Process_template  SystemSampleTime=-1  VariantActivationTime=update diagram  Latency=0  AutoFrameSizeCalculation=off
      link override debdec: Value=KINP_CANMsgInvalidGWZoneFR2_flg_debdec
      link override debinc: Value=KINP_CANMsgInvalidGWZoneFR2_flg_debinc
      link override deblim: Value=KINP_CANMsgInvalidGWZoneFR2_flg_deblim
      link override inverse: Value=KINP_CANMsgInvalidGWZoneFR2_flg_inverse
      link override ovrdflg: Value=KINP_CANMsgInvalidGWZoneFR2_flg_ovrdflg
      link override ovrdval: Value=KINP_CANMsgInvalidGWZoneFR2_flg_ovrdval
      link override srvcflg: Value=KINP_CANMsgInvalidGWZoneFR2_flg_srvcflg
      link override srvcval: Value=KINP_CANMsgInvalidGWZoneFR2_flg_srvcval
  CANMsgInvalidZoneDrSCP : FVT_lib/inp/CAN_Msg_Validity_Process_template  SystemSampleTime=-1  VariantActivationTime=update diagram  Latency=0  AutoFrameSizeCalculation=off
      link override debdec: Value=KINP_CANMsgInvalidZoneDrSCP_flg_debdec
      link override debinc: Value=KINP_CANMsgInvalidZoneDrSCP_flg_debinc
      link override deblim: Value=KINP_CANMsgInvalidZoneDrSCP_flg_deblim
      link override inverse: Value=KINP_CANMsgInvalidZoneDrSCP_flg_inverse
      link override ovrdflg: Value=KINP_CANMsgInvalidZoneDrSCP_flg_ovrdflg
      link override ovrdval: Value=KINP_CANMsgInvalidZoneDrSCP_flg_ovrdval
      link override srvcflg: Value=KINP_CANMsgInvalidZoneDrSCP_flg_srvcflg
      link override srvcval: Value=KINP_CANMsgInvalidZoneDrSCP_flg_srvcval
  CANMsgInvalidZoneDrTHCM : FVT_lib/inp/CAN_Msg_Validity_Process_template  SystemSampleTime=-1  VariantActivationTime=update diagram  Latency=0  AutoFrameSizeCalculation=off
      link override debdec: Value=KINP_CANMsgInvalidZoneDrTHCM_flg_debdec
      link override debinc: Value=KINP_CANMsgInvalidZoneDrTHCM_flg_debinc
      link override deblim: Value=KINP_CANMsgInvalidZoneDrTHCM_flg_deblim
      link override inverse: Value=KINP_CANMsgInvalidZoneDrTHCM_flg_inverse
      link override ovrdflg: Value=KINP_CANMsgInvalidZoneDrTHCM_flg_ovrdflg
      link override ovrdval: Value=KINP_CANMsgInvalidZoneDrTHCM_flg_ovrdval
      link override srvcflg: Value=KINP_CANMsgInvalidZoneDrTHCM_flg_srvcflg
      link override srvcval: Value=KINP_CANMsgInvalidZoneDrTHCM_flg_srvcval
  CANMsgInvalidZoneDrVCU : FVT_lib/inp/CAN_Msg_Validity_Process_template  SystemSampleTime=-1  VariantActivationTime=update diagram  Latency=0  AutoFrameSizeCalculation=off
      link override debdec: Value=KINP_CANMsgInvalidZoneDrVCU_flg_debdec
      link override debinc: Value=KINP_CANMsgInvalidZoneDrVCU_flg_debinc
      link override deblim: Value=KINP_CANMsgInvalidZoneDrVCU_flg_deblim
      link override inverse: Value=KINP_CANMsgInvalidZoneDrVCU_flg_inverse
      link override ovrdflg: Value=KINP_CANMsgInvalidZoneDrVCU_flg_ovrdflg
      link override ovrdval: Value=KINP_CANMsgInvalidZoneDrVCU_flg_ovrdval
      link override srvcflg: Value=KINP_CANMsgInvalidZoneDrVCU_flg_srvcflg
      link override srvcval: Value=KINP_CANMsgInvalidZoneDrVCU_flg_srvcval
  CANMsgInvalidZoneFrTHCM : FVT_lib/inp/CAN_Msg_Validity_Process_template  SystemSampleTime=-1  VariantActivationTime=update diagram  Latency=0  AutoFrameSizeCalculation=off
      link override debdec: Value=KINP_CANMsgInvalidZoneFrTHCM_flg_debdec
      link override debinc: Value=KINP_CANMsgInvalidZoneFrTHCM_flg_debinc
      link override deblim: Value=KINP_CANMsgInvalidZoneFrTHCM_flg_deblim
      link override inverse: Value=KINP_CANMsgInvalidZoneFrTHCM_flg_inverse
      link override ovrdflg: Value=KINP_CANMsgInvalidZoneFrTHCM_flg_ovrdflg
      link override ovrdval: Value=KINP_CANMsgInvalidZoneFrTHCM_flg_ovrdval
      link override srvcflg: Value=KINP_CANMsgInvalidZoneFrTHCM_flg_srvcflg
      link override srvcval: Value=KINP_CANMsgInvalidZoneFrTHCM_flg_srvcval
  bus_creator : BusCreator  Inputs=14
  bus_selector : BusSelector  OutputSignals=VHAL_CANMsgInvalidDKC1_flg,VHAL_CANMsgInvalidDKC2_flg,VHAL_CANMsgInvalidGWZDRPTG1_flg,VHAL_CANMsgInvalidGWZoneDR1_flg,VHAL_CANMsgInvalidGWZoneDR2_flg,VHAL_CANMsgInvalidGWZoneDR3_flg,VHAL_CANMsgInvalidGWZoneDR4_flg,VHAL_CANMsgInvalidGWZoneDR6_flg,VHAL_CANMsgInvalidGWZoneFR1_flg,VHAL_CANMsgInvalidGWZoneFR2_flg,VHAL_CANMsgInvalidZoneDrSCP_flg,VHAL_CANMsgInvalidZoneDrTHCM_flg,VHAL_CANMsgInvalidZoneDrVCU_flg,VHAL_CANMsgInvalidZoneFrTHCM_flg
  not{1..14} (14 alike) : Logic  Operator=NOT  AllPortsSameDT=off  OutDataTypeStr=boolean
  inp_CanValid_bus : Outport
  wires:
  BHAL_outputs/1 -> [BHAL_outputs]
  bus_selector/1 -> CANMsgInvalidDKC1/1  "<VHAL_CANMsgInvalidDKC1_flg>"
  CANMsgInvalidDKC1/1 -> not1/1
  not1/1 -> bus_creator/1  "VINP_CANMsgValidDKC1_flg"
  bus_selector/2 -> CANMsgInvalidDKC2/1  "<VHAL_CANMsgInvalidDKC2_flg>"
  CANMsgInvalidDKC2/1 -> not2/1
  not2/1 -> bus_creator/2  "VINP_CANMsgValidDKC2_flg"
  bus_selector/3 -> CANMsgInvalidGWZDRPTG1/1  "<VHAL_CANMsgInvalidGWZDRPTG1_flg>"
  CANMsgInvalidGWZDRPTG1/1 -> not3/1
  not3/1 -> bus_creator/3  "VINP_CANMsgValidGWZDRPTG1_flg"
  bus_selector/4 -> CANMsgInvalidGWZoneDR1/1  "<VHAL_CANMsgInvalidGWZoneDR1_flg>"
  CANMsgInvalidGWZoneDR1/1 -> not4/1
  not4/1 -> bus_creator/4  "VINP_CANMsgValidGWZoneDR1_flg"
  bus_selector/5 -> CANMsgInvalidGWZoneDR2/1  "<VHAL_CANMsgInvalidGWZoneDR2_flg>"
  CANMsgInvalidGWZoneDR2/1 -> not5/1
  not5/1 -> bus_creator/5  "VINP_CANMsgValidGWZoneDR2_flg"
  bus_selector/6 -> CANMsgInvalidGWZoneDR3/1  "<VHAL_CANMsgInvalidGWZoneDR3_flg>"
  CANMsgInvalidGWZoneDR3/1 -> not6/1
  not6/1 -> bus_creator/6  "VINP_CANMsgValidGWZoneDR3_flg"
  bus_selector/7 -> CANMsgInvalidGWZoneDR4/1  "<VHAL_CANMsgInvalidGWZoneDR4_flg>"
  CANMsgInvalidGWZoneDR4/1 -> not7/1
  not7/1 -> bus_creator/7  "VINP_CANMsgValidGWZoneDR4_flg"
  bus_selector/8 -> CANMsgInvalidGWZoneDR6/1  "<VHAL_CANMsgInvalidGWZoneDR6_flg>"
  CANMsgInvalidGWZoneDR6/1 -> not8/1
  not8/1 -> bus_creator/8  "VINP_CANMsgValidGWZoneDR6_flg"
  bus_selector/9 -> CANMsgInvalidGWZoneFR1/1  "<VHAL_CANMsgInvalidGWZoneFR1_flg>"
  CANMsgInvalidGWZoneFR1/1 -> not9/1
  not9/1 -> bus_creator/9  "VINP_CANMsgValidGWZoneFR1_flg"
  bus_selector/10 -> CANMsgInvalidGWZoneFR2/1  "<VHAL_CANMsgInvalidGWZoneFR2_flg>"
  CANMsgInvalidGWZoneFR2/1 -> not10/1
  not10/1 -> bus_creator/10  "VINP_CANMsgValidGWZoneFR2_flg"
  bus_selector/11 -> CANMsgInvalidZoneDrSCP/1  "<VHAL_CANMsgInvalidZoneDrSCP_flg>"
  CANMsgInvalidZoneDrSCP/1 -> not11/1
  not11/1 -> bus_creator/11  "VINP_CANMsgValidZoneDrSCP_flg"
  bus_selector/12 -> CANMsgInvalidZoneDrTHCM/1  "<VHAL_CANMsgInvalidZoneDrTHCM_flg>"
  CANMsgInvalidZoneDrTHCM/1 -> not12/1
  not12/1 -> bus_creator/12  "VINP_CANMsgValidZoneDrTHCM_flg"
  bus_selector/13 -> CANMsgInvalidZoneDrVCU/1  "<VHAL_CANMsgInvalidZoneDrVCU_flg>"
  CANMsgInvalidZoneDrVCU/1 -> not13/1
  not13/1 -> bus_creator/13  "VINP_CANMsgValidZoneDrVCU_flg"
  bus_selector/14 -> CANMsgInvalidZoneFrTHCM/1  "<VHAL_CANMsgInvalidZoneFrTHCM_flg>"
  CANMsgInvalidZoneFrTHCM/1 -> not14/1
  not14/1 -> bus_creator/14  "VINP_CANMsgValidZoneFrTHCM_flg"
  [BHAL_outputs] -> bus_selector/1
  bus_creator/1 -> inp_CanValid_bus/1
